simulink model "PART2"  (R2018b)
settings: Solver=ode2  StartTime=0.0  StopTime=500  FixedStep=0.1  RelTol=1e-3
settings Model: Creator=HP  LastModifiedBy=swastik

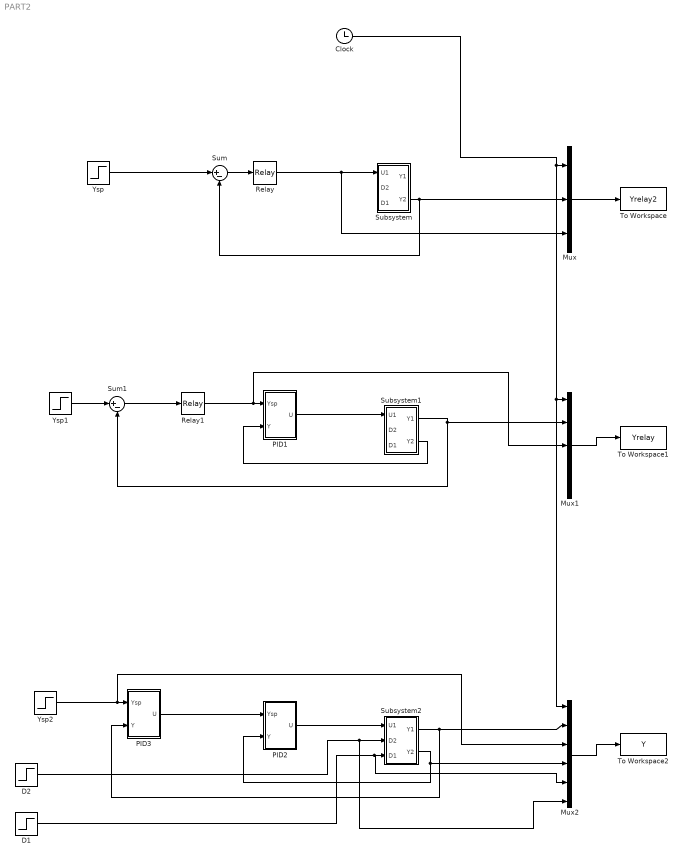
== system PART2 ==
  Clock : Clock
  D1 : Step  Time=0  After=0  SampleTime=0
  D2 : Step  Time=0  SampleTime=0
  Mux : Mux  Inputs=3
  Mux1 : Mux  Inputs=5
  Mux2 : Mux  Inputs=6
  PID1 : Subsystem  mask{Kc=1.6804/1.7, Ti=31.9/2, Td=31.9/8}
      mask prompts: Kc "Proportional Gain"; Ti "Integral time"; Td "Derivative time"
  PID2 : Subsystem  mask{Kc=1.6804/1.7, Ti=31.9/2, Td=31.9/8}
      mask prompts: Kc "Proportional Gain"; Ti "Integral time"; Td "Derivative time"
  PID3 : Subsystem  mask{Kc=2.0073/1.7, Ti=89.1/2, Td=89.1/8}
      mask prompts: Kc "Proportional Gain"; Ti "Integral time"; Td "Derivative time"
  Relay : Relay  OffOutputValue=-1
  Relay1 : Relay  OffOutputValue=-1
  Subsystem : Subsystem
  Subsystem1 : Subsystem
  Subsystem2 : Subsystem
  Sum : Sum  Inputs=|+-
  Sum1 : Sum  Inputs=|+-
  To Workspace : ToWorkspace  VariableName=Yrelay2  SampleTime=-1
  To Workspace1 : ToWorkspace  VariableName=Yrelay  SampleTime=-1
  To Workspace2 : ToWorkspace  VariableName=Y  SampleTime=-1
  Ysp : Step  Time=0  After=0  SampleTime=0
  Ysp1 : Step  Time=0  After=0  SampleTime=0
  Ysp2 : Step  Time=0  After=0  SampleTime=0
  wires:
  Ysp/1 -> Sum/1
  Sum/1 -> Relay/1
  Relay/1 -> Subsystem/1(U1), Mux/3
  Mux/1 -> To Workspace/1
  Clock/1 -> Mux2/1, Mux1/1, Mux/1
  Mux1/1 -> To Workspace1/1
  Subsystem/2(Y2) -> Mux/2, Sum/2
  PID1/1(U) -> Subsystem1/1(U1)
  Subsystem1/2(Y2) -> PID1/2(Y)
  Relay1/1 -> Mux1/3, PID1/1(Ysp)
  Sum1/1 -> Relay1/1
  Ysp1/1 -> Sum1/1
  Subsystem1/1(Y1) -> Mux1/2, Sum1/2
  Mux2/1 -> To Workspace2/1
  Subsystem2/2(Y2) -> Mux2/4, PID2/2(Y)
  PID2/1(U) -> Subsystem2/1(U1)
  Subsystem2/1(Y1) -> Mux2/2, PID3/2(Y)
  PID3/1(U) -> PID2/1(Ysp)
  Ysp2/1 -> Mux2/3, PID3/1(Ysp)
  D1/1 -> Mux2/5, Subsystem2/3(D1)
  D2/1 -> Mux2/6, Subsystem2/2(D2)

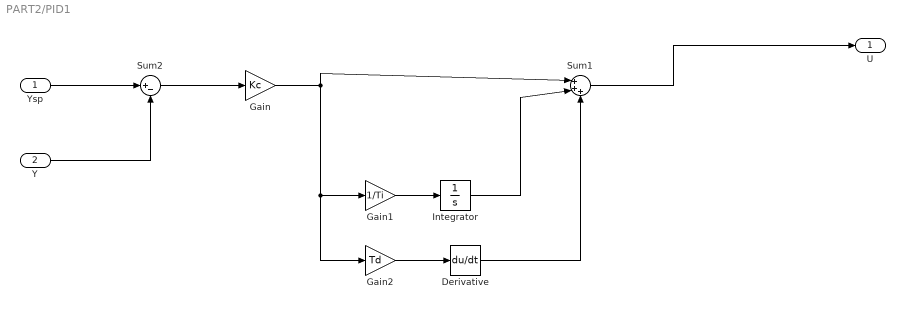
== system PART2/PID1 ==
  Ysp : Inport
  Y : Inport  Port=2
  Derivative : Derivative
  Gain : Gain  Gain=Kc
  Gain1 : Gain  Gain=1/Ti
  Gain2 : Gain  Gain=Td
  Integrator : Integrator
  Sum1 : Sum  Inputs=|+++
  Sum2 : Sum  Inputs=|+-
  U : Outport
  wires:
  Integrator/1 -> Sum1/2
  Gain/1 -> Sum1/1, Gain1/1, Gain2/1
  Sum2/1 -> Gain/1
  Y/1 -> Sum2/2
  Gain1/1 -> Integrator/1
  Gain2/1 -> Derivative/1
  Derivative/1 -> Sum1/3
  Ysp/1 -> Sum2/1
  Sum1/1 -> U/1

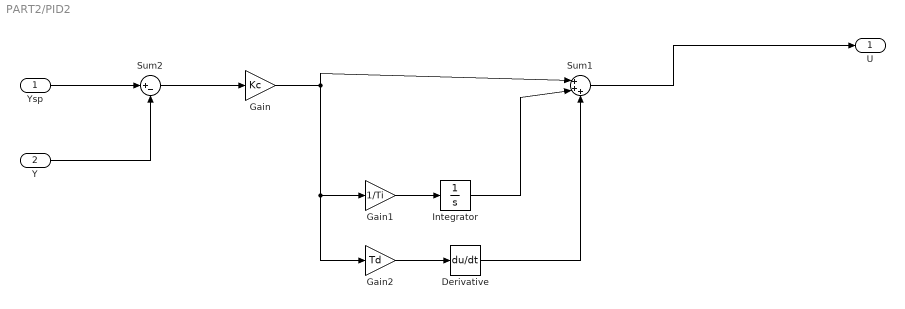
== system PART2/PID2 ==
  Ysp : Inport
  Y : Inport  Port=2
  Derivative : Derivative
  Gain : Gain  Gain=Kc
  Gain1 : Gain  Gain=1/Ti
  Gain2 : Gain  Gain=Td
  Integrator : Integrator
  Sum1 : Sum  Inputs=|+++
  Sum2 : Sum  Inputs=|+-
  U : Outport
  wires:
  Integrator/1 -> Sum1/2
  Gain/1 -> Sum1/1, Gain1/1, Gain2/1
  Sum2/1 -> Gain/1
  Y/1 -> Sum2/2
  Gain1/1 -> Integrator/1
  Gain2/1 -> Derivative/1
  Derivative/1 -> Sum1/3
  Ysp/1 -> Sum2/1
  Sum1/1 -> U/1

== system PART2/PID3 ==
  Ysp : Inport
  Y : Inport  Port=2
  Derivative : Derivative
  Gain : Gain  Gain=Kc
  Gain1 : Gain  Gain=1/Ti
  Gain2 : Gain  Gain=Td
  Integrator : Integrator
  Sum1 : Sum  Inputs=|+++
  Sum2 : Sum  Inputs=|+-
  U : Outport
  wires:
  Integrator/1 -> Sum1/2
  Gain/1 -> Sum1/1, Gain1/1, Gain2/1
  Sum2/1 -> Gain/1
  Y/1 -> Sum2/2
  Gain1/1 -> Integrator/1
  Gain2/1 -> Derivative/1
  Derivative/1 -> Sum1/3
  Ysp/1 -> Sum2/1
  Sum1/1 -> U/1

== system PART2/Subsystem ==
  U1 : Inport
  D2 : Inport  Port=2
  D1 : Inport  Port=3
  Process : Subsystem
  Y1 : Outport
  Y2 : Outport  Port=2
  wires:
  U1/1 -> Process/1(U)
  D2/1 -> Process/2(D2)
  D1/1 -> Process/3(D1)
  Process/1(Y1) -> Y1/1
  Process/2(Y2) -> Y2/1

== system PART2/Subsystem1 ==
  U1 : Inport
  D2 : Inport  Port=2
  D1 : Inport  Port=3
  Process : Subsystem
  Y1 : Outport
  Y2 : Outport  Port=2
  wires:
  U1/1 -> Process/1(U)
  D2/1 -> Process/2(D2)
  D1/1 -> Process/3(D1)
  Process/1(Y1) -> Y1/1
  Process/2(Y2) -> Y2/1

== system PART2/Subsystem2 ==
  U1 : Inport
  D2 : Inport  Port=2
  D1 : Inport  Port=3
  Process : Subsystem
  Y1 : Outport
  Y2 : Outport  Port=2
  wires:
  U1/1 -> Process/1(U)
  D2/1 -> Process/2(D2)
  D1/1 -> Process/3(D1)
  Process/1(Y1) -> Y1/1
  Process/2(Y2) -> Y2/1

== system PART2/Subsystem/Process ==
  U : Inport
  D2 : Inport  Port=2
  D1 : Inport  Port=3
  G1 : Subsystem  mask{K1=0.45, K2=0.45, T1=0.3, T2=0.3, K=1/17e-4}
      mask prompts: K1 "Forward Gain"; K2 "Rev Gain"; T1 "Forward Time Constt"; T2 "Rev Time Constt"; K "Scaling Gain"
  G2 : Subsystem  mask{K1=0.45, K2=0.45, T1=0.15, T2=0.15, K=2.01/17e-4}
      mask prompts: K1 "Forward Gain"; K2 "Rev Gain"; T1 "Forward Time Constt"; T2 "Rev Time Constt"; K "Scaling Gain"
  GD1 : Subsystem  mask{K1=0.45, K2=0.45, T1=0.1, T2=0.1, K=-1.005/17e-4}
      mask prompts: K1 "Forward Gain"; K2 "Rev Gain"; T1 "Forward Time Constt"; T2 "Rev Time Constt"; K "Scaling Gain"
  Sum : Sum  Inputs=|++
  Sum1 : Sum  Inputs=|++
  Y1 : Outport
  Y2 : Outport  Port=2
  wires:
  G1/1(Y) -> Sum1/1
  Sum/1 -> Y2/1, G1/1(U)
  G2/1(Y) -> Sum/1
  GD1/1(Y) -> Sum1/2
  U/1 -> G2/1(U)
  D1/1 -> GD1/1(U)
  D2/1 -> Sum/2
  Sum1/1 -> Y1/1

== system PART2/Subsystem1/Process ==
  U : Inport
  D2 : Inport  Port=2
  D1 : Inport  Port=3
  G1 : Subsystem  mask{K1=0.45, K2=0.45, T1=0.3, T2=0.3, K=1/17e-4}
      mask prompts: K1 "Forward Gain"; K2 "Rev Gain"; T1 "Forward Time Constt"; T2 "Rev Time Constt"; K "Scaling Gain"
  G2 : Subsystem  mask{K1=0.45, K2=0.45, T1=0.15, T2=0.15, K=2.01/17e-4}
      mask prompts: K1 "Forward Gain"; K2 "Rev Gain"; T1 "Forward Time Constt"; T2 "Rev Time Constt"; K "Scaling Gain"
  GD1 : Subsystem  mask{K1=0.45, K2=0.45, T1=0.1, T2=0.1, K=-1.005/17e-4}
      mask prompts: K1 "Forward Gain"; K2 "Rev Gain"; T1 "Forward Time Constt"; T2 "Rev Time Constt"; K "Scaling Gain"
  Sum : Sum  Inputs=|++
  Sum1 : Sum  Inputs=|++
  Y1 : Outport
  Y2 : Outport  Port=2
  wires:
  G1/1(Y) -> Sum1/1
  Sum/1 -> Y2/1, G1/1(U)
  G2/1(Y) -> Sum/1
  GD1/1(Y) -> Sum1/2
  U/1 -> G2/1(U)
  D1/1 -> GD1/1(U)
  D2/1 -> Sum/2
  Sum1/1 -> Y1/1

== system PART2/Subsystem2/Process ==
  U : Inport
  D2 : Inport  Port=2
  D1 : Inport  Port=3
  G1 : Subsystem  mask{K1=0.45, K2=0.45, T1=0.3, T2=0.3, K=1/17e-4}
      mask prompts: K1 "Forward Gain"; K2 "Rev Gain"; T1 "Forward Time Constt"; T2 "Rev Time Constt"; K "Scaling Gain"
  G2 : Subsystem  mask{K1=0.45, K2=0.45, T1=0.15, T2=0.15, K=2.01/17e-4}
      mask prompts: K1 "Forward Gain"; K2 "Rev Gain"; T1 "Forward Time Constt"; T2 "Rev Time Constt"; K "Scaling Gain"
  GD1 : Subsystem  mask{K1=0.45, K2=0.45, T1=0.1, T2=0.1, K=-1.005/17e-4}
      mask prompts: K1 "Forward Gain"; K2 "Rev Gain"; T1 "Forward Time Constt"; T2 "Rev Time Constt"; K "Scaling Gain"
  Sum : Sum  Inputs=|++
  Sum1 : Sum  Inputs=|++
  Y1 : Outport
  Y2 : Outport  Port=2
  wires:
  G1/1(Y) -> Sum1/1
  Sum/1 -> Y2/1, G1/1(U)
  G2/1(Y) -> Sum/1
  GD1/1(Y) -> Sum1/2
  U/1 -> G2/1(U)
  D1/1 -> GD1/1(U)
  D2/1 -> Sum/2
  Sum1/1 -> Y1/1

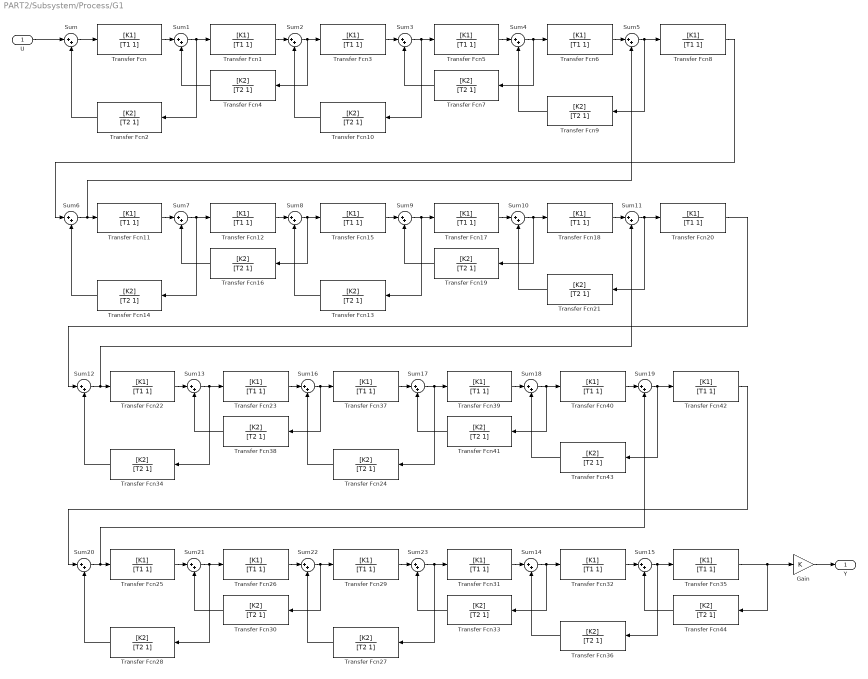
== system PART2/Subsystem/Process/G1 ==
  U : Inport
  Gain : Gain  Gain=K
  Sum{,1..23} (24 alike) : Sum  Inputs=|++
  Transfer Fcn{,1,3,5..6,8,11..12,15,17..18,20,22..23,25..26,29,31..32,35,37,39..40,42} (24 alike) : TransferFcn  Numerator=[K1]  Denominator=[T1 1]
  Transfer Fcn{2,4,7,9..10,13..14,16,19,21,24,27..28,30,33..34,36,38,41,43..44} (21 alike) : TransferFcn  Numerator=[K2]  Denominator=[T2 1]
  Y : Outport
  wires:
  Transfer Fcn14/1 -> Sum6/2
  Transfer Fcn13/1 -> Sum8/2
  Transfer Fcn18/1 -> Sum11/1
  Transfer Fcn1/1 -> Sum2/1
  Sum18/1 -> Transfer Fcn41/1, Transfer Fcn40/1
  Sum21/1 -> Transfer Fcn28/1, Transfer Fcn26/1
  Transfer Fcn26/1 -> Sum22/1
  Transfer Fcn15/1 -> Sum9/1
  Sum13/1 -> Transfer Fcn34/1, Transfer Fcn23/1
  Sum7/1 -> Transfer Fcn14/1, Transfer Fcn12/1
  Sum8/1 -> Transfer Fcn16/1, Transfer Fcn15/1
  Transfer Fcn20/1 -> Sum12/1
  Sum20/1 -> Sum19/2, Transfer Fcn25/1
  Transfer Fcn9/1 -> Sum4/2
  Transfer Fcn25/1 -> Sum21/1
  Sum12/1 -> Sum11/2, Transfer Fcn22/1
  Transfer Fcn12/1 -> Sum8/1
  Transfer Fcn16/1 -> Sum7/2
  Transfer Fcn44/1 -> Sum15/2
  Transfer Fcn39/1 -> Sum18/1
  Sum2/1 -> Transfer Fcn4/1, Transfer Fcn3/1
  Transfer Fcn38/1 -> Sum13/2
  Sum17/1 -> Transfer Fcn24/1, Transfer Fcn39/1
  Sum9/1 -> Transfer Fcn13/1, Transfer Fcn17/1
  Transfer Fcn35/1 -> Gain/1, Transfer Fcn44/1
  Sum11/1 -> Transfer Fcn21/1, Transfer Fcn20/1
  Transfer Fcn42/1 -> Sum20/1
  Sum1/1 -> Transfer Fcn2/1, Transfer Fcn1/1
  Sum15/1 -> Transfer Fcn36/1, Transfer Fcn35/1
  Transfer Fcn27/1 -> Sum22/2
  Transfer Fcn24/1 -> Sum16/2
  Transfer Fcn31/1 -> Sum14/1
  Transfer Fcn23/1 -> Sum16/1
  Sum14/1 -> Transfer Fcn33/1, Transfer Fcn32/1
  Sum23/1 -> Transfer Fcn27/1, Transfer Fcn31/1
  Transfer Fcn40/1 -> Sum19/1
  Sum16/1 -> Transfer Fcn38/1, Transfer Fcn37/1
  Transfer Fcn22/1 -> Sum13/1
  Transfer Fcn34/1 -> Sum12/2
  Transfer Fcn37/1 -> Sum17/1
  Transfer Fcn33/1 -> Sum23/2
  Transfer Fcn41/1 -> Sum17/2
  Sum4/1 -> Transfer Fcn7/1, Transfer Fcn6/1
  Transfer Fcn36/1 -> Sum14/2
  Sum10/1 -> Transfer Fcn19/1, Transfer Fcn18/1
  Sum22/1 -> Transfer Fcn30/1, Transfer Fcn29/1
  Transfer Fcn6/1 -> Sum5/1
  Transfer Fcn29/1 -> Sum23/1
  Transfer Fcn2/1 -> Sum/2
  Transfer Fcn28/1 -> Sum20/2
  Transfer Fcn17/1 -> Sum10/1
  Transfer Fcn30/1 -> Sum21/2
  Transfer Fcn43/1 -> Sum18/2
  Transfer Fcn5/1 -> Sum4/1
  Sum19/1 -> Transfer Fcn43/1, Transfer Fcn42/1
  Sum3/1 -> Transfer Fcn10/1, Transfer Fcn5/1
  Transfer Fcn32/1 -> Sum15/1
  Sum6/1 -> Sum5/2, Transfer Fcn11/1
  Transfer Fcn/1 -> Sum1/1
  Transfer Fcn21/1 -> Sum10/2
  Sum5/1 -> Transfer Fcn9/1, Transfer Fcn8/1
  Transfer Fcn7/1 -> Sum3/2
  Transfer Fcn4/1 -> Sum1/2
  Transfer Fcn11/1 -> Sum7/1
  Transfer Fcn10/1 -> Sum2/2
  Transfer Fcn3/1 -> Sum3/1
  Transfer Fcn8/1 -> Sum6/1
  Transfer Fcn19/1 -> Sum9/2
  Sum/1 -> Transfer Fcn/1
  Gain/1 -> Y/1
  U/1 -> Sum/1

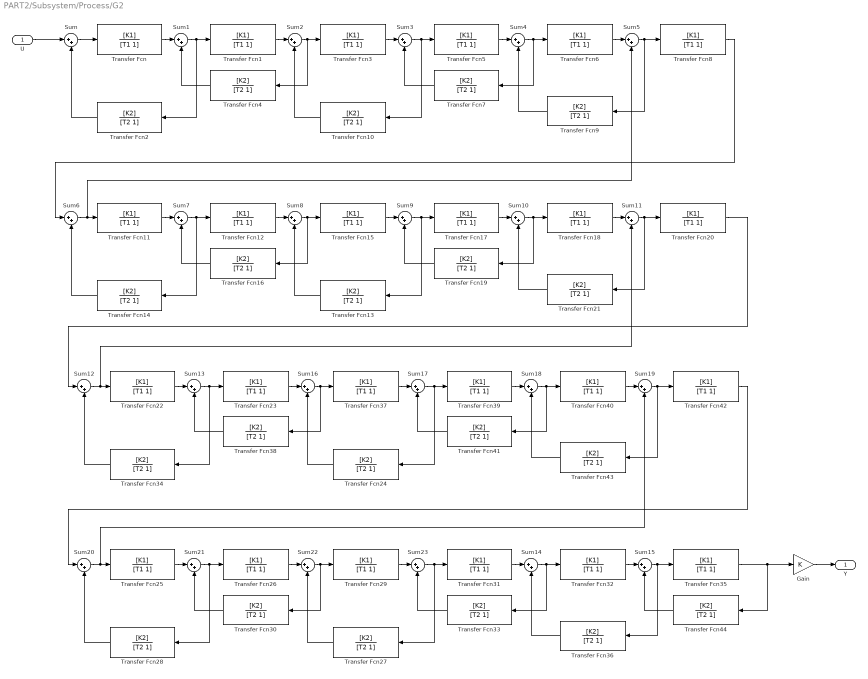
== system PART2/Subsystem/Process/G2 ==
  U : Inport
  Gain : Gain  Gain=K
  Sum{,1..23} (24 alike) : Sum  Inputs=|++
  Transfer Fcn{,1,3,5..6,8,11..12,15,17..18,20,22..23,25..26,29,31..32,35,37,39..40,42} (24 alike) : TransferFcn  Numerator=[K1]  Denominator=[T1 1]
  Transfer Fcn{2,4,7,9..10,13..14,16,19,21,24,27..28,30,33..34,36,38,41,43..44} (21 alike) : TransferFcn  Numerator=[K2]  Denominator=[T2 1]
  Y : Outport
  wires:
  Transfer Fcn14/1 -> Sum6/2
  Transfer Fcn13/1 -> Sum8/2
  Transfer Fcn18/1 -> Sum11/1
  Transfer Fcn1/1 -> Sum2/1
  Sum18/1 -> Transfer Fcn41/1, Transfer Fcn40/1
  Sum21/1 -> Transfer Fcn28/1, Transfer Fcn26/1
  Transfer Fcn26/1 -> Sum22/1
  Transfer Fcn15/1 -> Sum9/1
  Sum13/1 -> Transfer Fcn34/1, Transfer Fcn23/1
  Sum7/1 -> Transfer Fcn14/1, Transfer Fcn12/1
  Sum8/1 -> Transfer Fcn16/1, Transfer Fcn15/1
  Transfer Fcn20/1 -> Sum12/1
  Sum20/1 -> Sum19/2, Transfer Fcn25/1
  Transfer Fcn9/1 -> Sum4/2
  Transfer Fcn25/1 -> Sum21/1
  Sum12/1 -> Sum11/2, Transfer Fcn22/1
  Transfer Fcn12/1 -> Sum8/1
  Transfer Fcn16/1 -> Sum7/2
  Transfer Fcn44/1 -> Sum15/2
  Transfer Fcn39/1 -> Sum18/1
  Sum2/1 -> Transfer Fcn4/1, Transfer Fcn3/1
  Transfer Fcn38/1 -> Sum13/2
  Sum17/1 -> Transfer Fcn24/1, Transfer Fcn39/1
  Sum9/1 -> Transfer Fcn13/1, Transfer Fcn17/1
  Transfer Fcn35/1 -> Gain/1, Transfer Fcn44/1
  Sum11/1 -> Transfer Fcn21/1, Transfer Fcn20/1
  Transfer Fcn42/1 -> Sum20/1
  Sum1/1 -> Transfer Fcn2/1, Transfer Fcn1/1
  Sum15/1 -> Transfer Fcn36/1, Transfer Fcn35/1
  Transfer Fcn27/1 -> Sum22/2
  Transfer Fcn24/1 -> Sum16/2
  Transfer Fcn31/1 -> Sum14/1
  Transfer Fcn23/1 -> Sum16/1
  Sum14/1 -> Transfer Fcn33/1, Transfer Fcn32/1
  Sum23/1 -> Transfer Fcn27/1, Transfer Fcn31/1
  Transfer Fcn40/1 -> Sum19/1
  Sum16/1 -> Transfer Fcn38/1, Transfer Fcn37/1
  Transfer Fcn22/1 -> Sum13/1
  Transfer Fcn34/1 -> Sum12/2
  Transfer Fcn37/1 -> Sum17/1
  Transfer Fcn33/1 -> Sum23/2
  Transfer Fcn41/1 -> Sum17/2
  Sum4/1 -> Transfer Fcn7/1, Transfer Fcn6/1
  Transfer Fcn36/1 -> Sum14/2
  Sum10/1 -> Transfer Fcn19/1, Transfer Fcn18/1
  Sum22/1 -> Transfer Fcn30/1, Transfer Fcn29/1
  Transfer Fcn6/1 -> Sum5/1
  Transfer Fcn29/1 -> Sum23/1
  Transfer Fcn2/1 -> Sum/2
  Transfer Fcn28/1 -> Sum20/2
  Transfer Fcn17/1 -> Sum10/1
  Transfer Fcn30/1 -> Sum21/2
  Transfer Fcn43/1 -> Sum18/2
  Transfer Fcn5/1 -> Sum4/1
  Sum19/1 -> Transfer Fcn43/1, Transfer Fcn42/1
  Sum3/1 -> Transfer Fcn10/1, Transfer Fcn5/1
  Transfer Fcn32/1 -> Sum15/1
  Sum6/1 -> Sum5/2, Transfer Fcn11/1
  Transfer Fcn/1 -> Sum1/1
  Transfer Fcn21/1 -> Sum10/2
  Sum5/1 -> Transfer Fcn9/1, Transfer Fcn8/1
  Transfer Fcn7/1 -> Sum3/2
  Transfer Fcn4/1 -> Sum1/2
  Transfer Fcn11/1 -> Sum7/1
  Transfer Fcn10/1 -> Sum2/2
  Transfer Fcn3/1 -> Sum3/1
  Transfer Fcn8/1 -> Sum6/1
  Transfer Fcn19/1 -> Sum9/2
  Sum/1 -> Transfer Fcn/1
  Gain/1 -> Y/1
  U/1 -> Sum/1

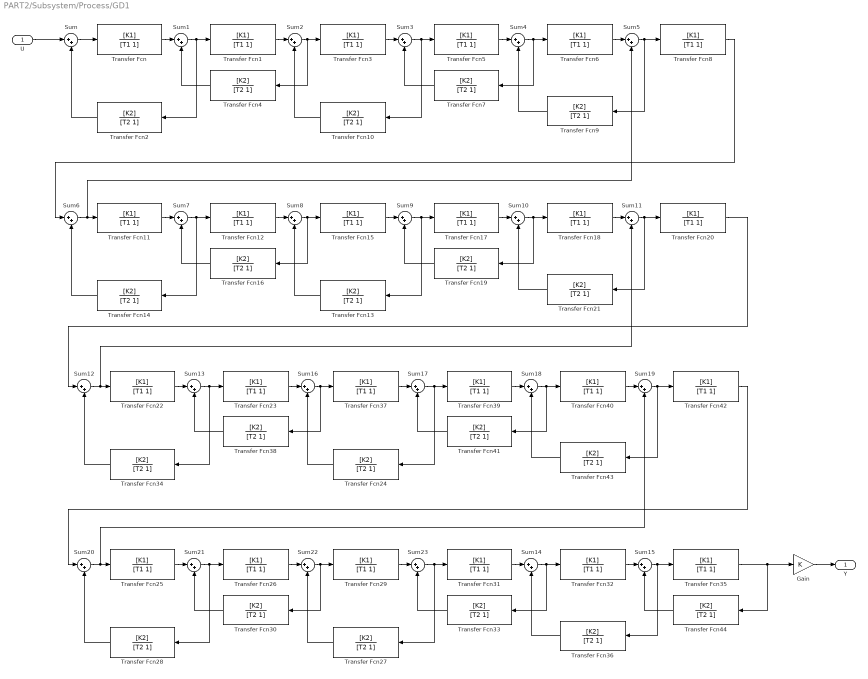
== system PART2/Subsystem/Process/GD1 ==
  U : Inport
  Gain : Gain  Gain=K
  Sum{,1..23} (24 alike) : Sum  Inputs=|++
  Transfer Fcn{,1,3,5..6,8,11..12,15,17..18,20,22..23,25..26,29,31..32,35,37,39..40,42} (24 alike) : TransferFcn  Numerator=[K1]  Denominator=[T1 1]
  Transfer Fcn{2,4,7,9..10,13..14,16,19,21,24,27..28,30,33..34,36,38,41,43..44} (21 alike) : TransferFcn  Numerator=[K2]  Denominator=[T2 1]
  Y : Outport
  wires:
  Transfer Fcn14/1 -> Sum6/2
  Transfer Fcn13/1 -> Sum8/2
  Transfer Fcn18/1 -> Sum11/1
  Transfer Fcn1/1 -> Sum2/1
  Sum18/1 -> Transfer Fcn41/1, Transfer Fcn40/1
  Sum21/1 -> Transfer Fcn28/1, Transfer Fcn26/1
  Transfer Fcn26/1 -> Sum22/1
  Transfer Fcn15/1 -> Sum9/1
  Sum13/1 -> Transfer Fcn34/1, Transfer Fcn23/1
  Sum7/1 -> Transfer Fcn14/1, Transfer Fcn12/1
  Sum8/1 -> Transfer Fcn16/1, Transfer Fcn15/1
  Transfer Fcn20/1 -> Sum12/1
  Sum20/1 -> Sum19/2, Transfer Fcn25/1
  Transfer Fcn9/1 -> Sum4/2
  Transfer Fcn25/1 -> Sum21/1
  Sum12/1 -> Sum11/2, Transfer Fcn22/1
  Transfer Fcn12/1 -> Sum8/1
  Transfer Fcn16/1 -> Sum7/2
  Transfer Fcn44/1 -> Sum15/2
  Transfer Fcn39/1 -> Sum18/1
  Sum2/1 -> Transfer Fcn4/1, Transfer Fcn3/1
  Transfer Fcn38/1 -> Sum13/2
  Sum17/1 -> Transfer Fcn24/1, Transfer Fcn39/1
  Sum9/1 -> Transfer Fcn13/1, Transfer Fcn17/1
  Transfer Fcn35/1 -> Gain/1, Transfer Fcn44/1
  Sum11/1 -> Transfer Fcn21/1, Transfer Fcn20/1
  Transfer Fcn42/1 -> Sum20/1
  Sum1/1 -> Transfer Fcn2/1, Transfer Fcn1/1
  Sum15/1 -> Transfer Fcn36/1, Transfer Fcn35/1
  Transfer Fcn27/1 -> Sum22/2
  Transfer Fcn24/1 -> Sum16/2
  Transfer Fcn31/1 -> Sum14/1
  Transfer Fcn23/1 -> Sum16/1
  Sum14/1 -> Transfer Fcn33/1, Transfer Fcn32/1
  Sum23/1 -> Transfer Fcn27/1, Transfer Fcn31/1
  Transfer Fcn40/1 -> Sum19/1
  Sum16/1 -> Transfer Fcn38/1, Transfer Fcn37/1
  Transfer Fcn22/1 -> Sum13/1
  Transfer Fcn34/1 -> Sum12/2
  Transfer Fcn37/1 -> Sum17/1
  Transfer Fcn33/1 -> Sum23/2
  Transfer Fcn41/1 -> Sum17/2
  Sum4/1 -> Transfer Fcn7/1, Transfer Fcn6/1
  Transfer Fcn36/1 -> Sum14/2
  Sum10/1 -> Transfer Fcn19/1, Transfer Fcn18/1
  Sum22/1 -> Transfer Fcn30/1, Transfer Fcn29/1
  Transfer Fcn6/1 -> Sum5/1
  Transfer Fcn29/1 -> Sum23/1
  Transfer Fcn2/1 -> Sum/2
  Transfer Fcn28/1 -> Sum20/2
  Transfer Fcn17/1 -> Sum10/1
  Transfer Fcn30/1 -> Sum21/2
  Transfer Fcn43/1 -> Sum18/2
  Transfer Fcn5/1 -> Sum4/1
  Sum19/1 -> Transfer Fcn43/1, Transfer Fcn42/1
  Sum3/1 -> Transfer Fcn10/1, Transfer Fcn5/1
  Transfer Fcn32/1 -> Sum15/1
  Sum6/1 -> Sum5/2, Transfer Fcn11/1
  Transfer Fcn/1 -> Sum1/1
  Transfer Fcn21/1 -> Sum10/2
  Sum5/1 -> Transfer Fcn9/1, Transfer Fcn8/1
  Transfer Fcn7/1 -> Sum3/2
  Transfer Fcn4/1 -> Sum1/2
  Transfer Fcn11/1 -> Sum7/1
  Transfer Fcn10/1 -> Sum2/2
  Transfer Fcn3/1 -> Sum3/1
  Transfer Fcn8/1 -> Sum6/1
  Transfer Fcn19/1 -> Sum9/2
  Sum/1 -> Transfer Fcn/1
  Gain/1 -> Y/1
  U/1 -> Sum/1

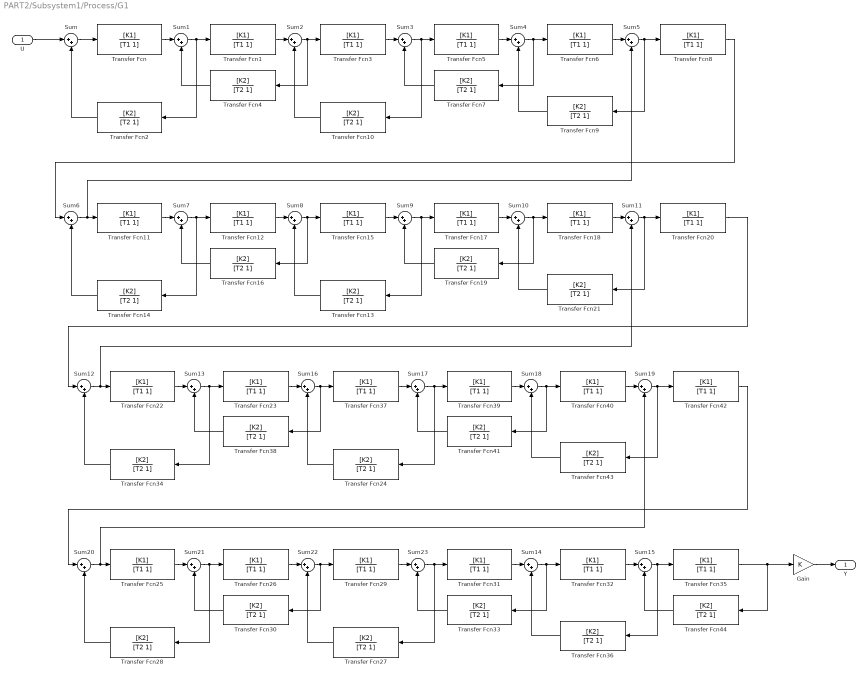
== system PART2/Subsystem1/Process/G1 ==
  U : Inport
  Gain : Gain  Gain=K
  Sum{,1..23} (24 alike) : Sum  Inputs=|++
  Transfer Fcn{,1,3,5..6,8,11..12,15,17..18,20,22..23,25..26,29,31..32,35,37,39..40,42} (24 alike) : TransferFcn  Numerator=[K1]  Denominator=[T1 1]
  Transfer Fcn{2,4,7,9..10,13..14,16,19,21,24,27..28,30,33..34,36,38,41,43..44} (21 alike) : TransferFcn  Numerator=[K2]  Denominator=[T2 1]
  Y : Outport
  wires:
  Transfer Fcn14/1 -> Sum6/2
  Transfer Fcn13/1 -> Sum8/2
  Transfer Fcn18/1 -> Sum11/1
  Transfer Fcn1/1 -> Sum2/1
  Sum18/1 -> Transfer Fcn41/1, Transfer Fcn40/1
  Sum21/1 -> Transfer Fcn28/1, Transfer Fcn26/1
  Transfer Fcn26/1 -> Sum22/1
  Transfer Fcn15/1 -> Sum9/1
  Sum13/1 -> Transfer Fcn34/1, Transfer Fcn23/1
  Sum7/1 -> Transfer Fcn14/1, Transfer Fcn12/1
  Sum8/1 -> Transfer Fcn16/1, Transfer Fcn15/1
  Transfer Fcn20/1 -> Sum12/1
  Sum20/1 -> Sum19/2, Transfer Fcn25/1
  Transfer Fcn9/1 -> Sum4/2
  Transfer Fcn25/1 -> Sum21/1
  Sum12/1 -> Sum11/2, Transfer Fcn22/1
  Transfer Fcn12/1 -> Sum8/1
  Transfer Fcn16/1 -> Sum7/2
  Transfer Fcn44/1 -> Sum15/2
  Transfer Fcn39/1 -> Sum18/1
  Sum2/1 -> Transfer Fcn4/1, Transfer Fcn3/1
  Transfer Fcn38/1 -> Sum13/2
  Sum17/1 -> Transfer Fcn24/1, Transfer Fcn39/1
  Sum9/1 -> Transfer Fcn13/1, Transfer Fcn17/1
  Transfer Fcn35/1 -> Gain/1, Transfer Fcn44/1
  Sum11/1 -> Transfer Fcn21/1, Transfer Fcn20/1
  Transfer Fcn42/1 -> Sum20/1
  Sum1/1 -> Transfer Fcn2/1, Transfer Fcn1/1
  Sum15/1 -> Transfer Fcn36/1, Transfer Fcn35/1
  Transfer Fcn27/1 -> Sum22/2
  Transfer Fcn24/1 -> Sum16/2
  Transfer Fcn31/1 -> Sum14/1
  Transfer Fcn23/1 -> Sum16/1
  Sum14/1 -> Transfer Fcn33/1, Transfer Fcn32/1
  Sum23/1 -> Transfer Fcn27/1, Transfer Fcn31/1
  Transfer Fcn40/1 -> Sum19/1
  Sum16/1 -> Transfer Fcn38/1, Transfer Fcn37/1
  Transfer Fcn22/1 -> Sum13/1
  Transfer Fcn34/1 -> Sum12/2
  Transfer Fcn37/1 -> Sum17/1
  Transfer Fcn33/1 -> Sum23/2
  Transfer Fcn41/1 -> Sum17/2
  Sum4/1 -> Transfer Fcn7/1, Transfer Fcn6/1
  Transfer Fcn36/1 -> Sum14/2
  Sum10/1 -> Transfer Fcn19/1, Transfer Fcn18/1
  Sum22/1 -> Transfer Fcn30/1, Transfer Fcn29/1
  Transfer Fcn6/1 -> Sum5/1
  Transfer Fcn29/1 -> Sum23/1
  Transfer Fcn2/1 -> Sum/2
  Transfer Fcn28/1 -> Sum20/2
  Transfer Fcn17/1 -> Sum10/1
  Transfer Fcn30/1 -> Sum21/2
  Transfer Fcn43/1 -> Sum18/2
  Transfer Fcn5/1 -> Sum4/1
  Sum19/1 -> Transfer Fcn43/1, Transfer Fcn42/1
  Sum3/1 -> Transfer Fcn10/1, Transfer Fcn5/1
  Transfer Fcn32/1 -> Sum15/1
  Sum6/1 -> Sum5/2, Transfer Fcn11/1
  Transfer Fcn/1 -> Sum1/1
  Transfer Fcn21/1 -> Sum10/2
  Sum5/1 -> Transfer Fcn9/1, Transfer Fcn8/1
  Transfer Fcn7/1 -> Sum3/2
  Transfer Fcn4/1 -> Sum1/2
  Transfer Fcn11/1 -> Sum7/1
  Transfer Fcn10/1 -> Sum2/2
  Transfer Fcn3/1 -> Sum3/1
  Transfer Fcn8/1 -> Sum6/1
  Transfer Fcn19/1 -> Sum9/2
  Sum/1 -> Transfer Fcn/1
  Gain/1 -> Y/1
  U/1 -> Sum/1

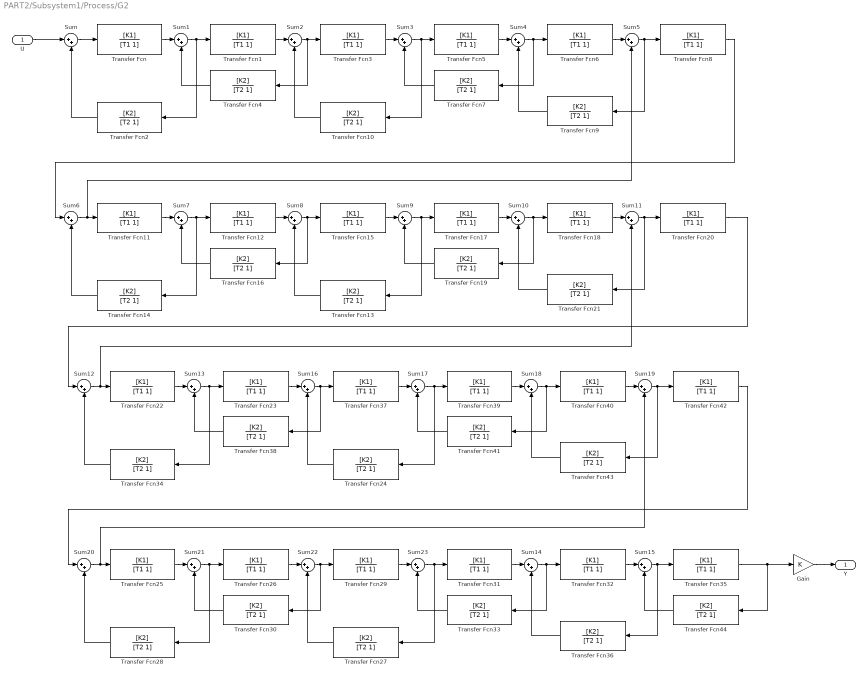
== system PART2/Subsystem1/Process/G2 ==
  U : Inport
  Gain : Gain  Gain=K
  Sum{,1..23} (24 alike) : Sum  Inputs=|++
  Transfer Fcn{,1,3,5..6,8,11..12,15,17..18,20,22..23,25..26,29,31..32,35,37,39..40,42} (24 alike) : TransferFcn  Numerator=[K1]  Denominator=[T1 1]
  Transfer Fcn{2,4,7,9..10,13..14,16,19,21,24,27..28,30,33..34,36,38,41,43..44} (21 alike) : TransferFcn  Numerator=[K2]  Denominator=[T2 1]
  Y : Outport
  wires:
  Transfer Fcn14/1 -> Sum6/2
  Transfer Fcn13/1 -> Sum8/2
  Transfer Fcn18/1 -> Sum11/1
  Transfer Fcn1/1 -> Sum2/1
  Sum18/1 -> Transfer Fcn41/1, Transfer Fcn40/1
  Sum21/1 -> Transfer Fcn28/1, Transfer Fcn26/1
  Transfer Fcn26/1 -> Sum22/1
  Transfer Fcn15/1 -> Sum9/1
  Sum13/1 -> Transfer Fcn34/1, Transfer Fcn23/1
  Sum7/1 -> Transfer Fcn14/1, Transfer Fcn12/1
  Sum8/1 -> Transfer Fcn16/1, Transfer Fcn15/1
  Transfer Fcn20/1 -> Sum12/1
  Sum20/1 -> Sum19/2, Transfer Fcn25/1
  Transfer Fcn9/1 -> Sum4/2
  Transfer Fcn25/1 -> Sum21/1
  Sum12/1 -> Sum11/2, Transfer Fcn22/1
  Transfer Fcn12/1 -> Sum8/1
  Transfer Fcn16/1 -> Sum7/2
  Transfer Fcn44/1 -> Sum15/2
  Transfer Fcn39/1 -> Sum18/1
  Sum2/1 -> Transfer Fcn4/1, Transfer Fcn3/1
  Transfer Fcn38/1 -> Sum13/2
  Sum17/1 -> Transfer Fcn24/1, Transfer Fcn39/1
  Sum9/1 -> Transfer Fcn13/1, Transfer Fcn17/1
  Transfer Fcn35/1 -> Gain/1, Transfer Fcn44/1
  Sum11/1 -> Transfer Fcn21/1, Transfer Fcn20/1
  Transfer Fcn42/1 -> Sum20/1
  Sum1/1 -> Transfer Fcn2/1, Transfer Fcn1/1
  Sum15/1 -> Transfer Fcn36/1, Transfer Fcn35/1
  Transfer Fcn27/1 -> Sum22/2
  Transfer Fcn24/1 -> Sum16/2
  Transfer Fcn31/1 -> Sum14/1
  Transfer Fcn23/1 -> Sum16/1
  Sum14/1 -> Transfer Fcn33/1, Transfer Fcn32/1
  Sum23/1 -> Transfer Fcn27/1, Transfer Fcn31/1
  Transfer Fcn40/1 -> Sum19/1
  Sum16/1 -> Transfer Fcn38/1, Transfer Fcn37/1
  Transfer Fcn22/1 -> Sum13/1
  Transfer Fcn34/1 -> Sum12/2
  Transfer Fcn37/1 -> Sum17/1
  Transfer Fcn33/1 -> Sum23/2
  Transfer Fcn41/1 -> Sum17/2
  Sum4/1 -> Transfer Fcn7/1, Transfer Fcn6/1
  Transfer Fcn36/1 -> Sum14/2
  Sum10/1 -> Transfer Fcn19/1, Transfer Fcn18/1
  Sum22/1 -> Transfer Fcn30/1, Transfer Fcn29/1
  Transfer Fcn6/1 -> Sum5/1
  Transfer Fcn29/1 -> Sum23/1
  Transfer Fcn2/1 -> Sum/2
  Transfer Fcn28/1 -> Sum20/2
  Transfer Fcn17/1 -> Sum10/1
  Transfer Fcn30/1 -> Sum21/2
  Transfer Fcn43/1 -> Sum18/2
  Transfer Fcn5/1 -> Sum4/1
  Sum19/1 -> Transfer Fcn43/1, Transfer Fcn42/1
  Sum3/1 -> Transfer Fcn10/1, Transfer Fcn5/1
  Transfer Fcn32/1 -> Sum15/1
  Sum6/1 -> Sum5/2, Transfer Fcn11/1
  Transfer Fcn/1 -> Sum1/1
  Transfer Fcn21/1 -> Sum10/2
  Sum5/1 -> Transfer Fcn9/1, Transfer Fcn8/1
  Transfer Fcn7/1 -> Sum3/2
  Transfer Fcn4/1 -> Sum1/2
  Transfer Fcn11/1 -> Sum7/1
  Transfer Fcn10/1 -> Sum2/2
  Transfer Fcn3/1 -> Sum3/1
  Transfer Fcn8/1 -> Sum6/1
  Transfer Fcn19/1 -> Sum9/2
  Sum/1 -> Transfer Fcn/1
  Gain/1 -> Y/1
  U/1 -> Sum/1

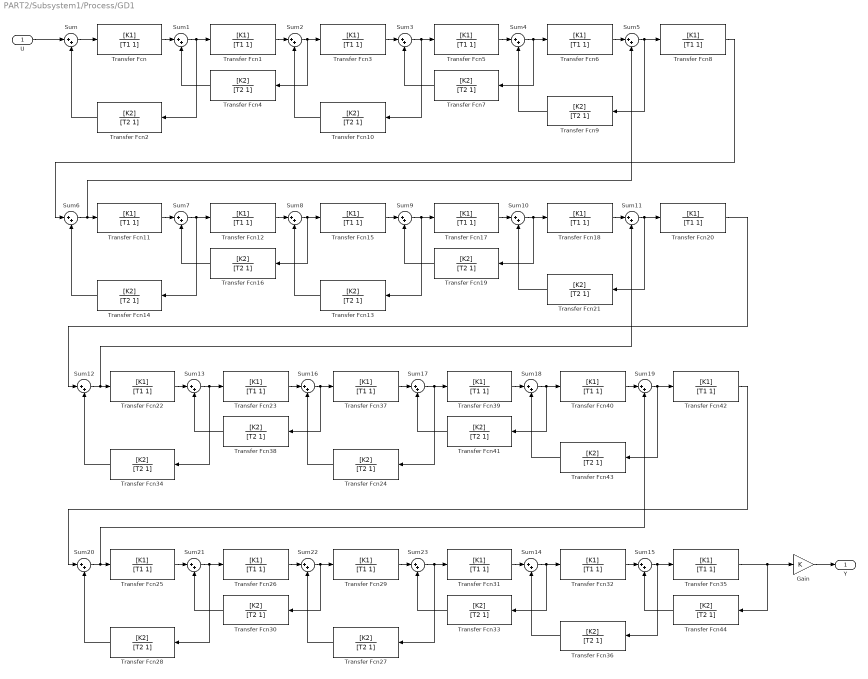
== system PART2/Subsystem1/Process/GD1 ==
  U : Inport
  Gain : Gain  Gain=K
  Sum{,1..23} (24 alike) : Sum  Inputs=|++
  Transfer Fcn{,1,3,5..6,8,11..12,15,17..18,20,22..23,25..26,29,31..32,35,37,39..40,42} (24 alike) : TransferFcn  Numerator=[K1]  Denominator=[T1 1]
  Transfer Fcn{2,4,7,9..10,13..14,16,19,21,24,27..28,30,33..34,36,38,41,43..44} (21 alike) : TransferFcn  Numerator=[K2]  Denominator=[T2 1]
  Y : Outport
  wires:
  Transfer Fcn14/1 -> Sum6/2
  Transfer Fcn13/1 -> Sum8/2
  Transfer Fcn18/1 -> Sum11/1
  Transfer Fcn1/1 -> Sum2/1
  Sum18/1 -> Transfer Fcn41/1, Transfer Fcn40/1
  Sum21/1 -> Transfer Fcn28/1, Transfer Fcn26/1
  Transfer Fcn26/1 -> Sum22/1
  Transfer Fcn15/1 -> Sum9/1
  Sum13/1 -> Transfer Fcn34/1, Transfer Fcn23/1
  Sum7/1 -> Transfer Fcn14/1, Transfer Fcn12/1
  Sum8/1 -> Transfer Fcn16/1, Transfer Fcn15/1
  Transfer Fcn20/1 -> Sum12/1
  Sum20/1 -> Sum19/2, Transfer Fcn25/1
  Transfer Fcn9/1 -> Sum4/2
  Transfer Fcn25/1 -> Sum21/1
  Sum12/1 -> Sum11/2, Transfer Fcn22/1
  Transfer Fcn12/1 -> Sum8/1
  Transfer Fcn16/1 -> Sum7/2
  Transfer Fcn44/1 -> Sum15/2
  Transfer Fcn39/1 -> Sum18/1
  Sum2/1 -> Transfer Fcn4/1, Transfer Fcn3/1
  Transfer Fcn38/1 -> Sum13/2
  Sum17/1 -> Transfer Fcn24/1, Transfer Fcn39/1
  Sum9/1 -> Transfer Fcn13/1, Transfer Fcn17/1
  Transfer Fcn35/1 -> Gain/1, Transfer Fcn44/1
  Sum11/1 -> Transfer Fcn21/1, Transfer Fcn20/1
  Transfer Fcn42/1 -> Sum20/1
  Sum1/1 -> Transfer Fcn2/1, Transfer Fcn1/1
  Sum15/1 -> Transfer Fcn36/1, Transfer Fcn35/1
  Transfer Fcn27/1 -> Sum22/2
  Transfer Fcn24/1 -> Sum16/2
  Transfer Fcn31/1 -> Sum14/1
  Transfer Fcn23/1 -> Sum16/1
  Sum14/1 -> Transfer Fcn33/1, Transfer Fcn32/1
  Sum23/1 -> Transfer Fcn27/1, Transfer Fcn31/1
  Transfer Fcn40/1 -> Sum19/1
  Sum16/1 -> Transfer Fcn38/1, Transfer Fcn37/1
  Transfer Fcn22/1 -> Sum13/1
  Transfer Fcn34/1 -> Sum12/2
  Transfer Fcn37/1 -> Sum17/1
  Transfer Fcn33/1 -> Sum23/2
  Transfer Fcn41/1 -> Sum17/2
  Sum4/1 -> Transfer Fcn7/1, Transfer Fcn6/1
  Transfer Fcn36/1 -> Sum14/2
  Sum10/1 -> Transfer Fcn19/1, Transfer Fcn18/1
  Sum22/1 -> Transfer Fcn30/1, Transfer Fcn29/1
  Transfer Fcn6/1 -> Sum5/1
  Transfer Fcn29/1 -> Sum23/1
  Transfer Fcn2/1 -> Sum/2
  Transfer Fcn28/1 -> Sum20/2
  Transfer Fcn17/1 -> Sum10/1
  Transfer Fcn30/1 -> Sum21/2
  Transfer Fcn43/1 -> Sum18/2
  Transfer Fcn5/1 -> Sum4/1
  Sum19/1 -> Transfer Fcn43/1, Transfer Fcn42/1
  Sum3/1 -> Transfer Fcn10/1, Transfer Fcn5/1
  Transfer Fcn32/1 -> Sum15/1
  Sum6/1 -> Sum5/2, Transfer Fcn11/1
  Transfer Fcn/1 -> Sum1/1
  Transfer Fcn21/1 -> Sum10/2
  Sum5/1 -> Transfer Fcn9/1, Transfer Fcn8/1
  Transfer Fcn7/1 -> Sum3/2
  Transfer Fcn4/1 -> Sum1/2
  Transfer Fcn11/1 -> Sum7/1
  Transfer Fcn10/1 -> Sum2/2
  Transfer Fcn3/1 -> Sum3/1
  Transfer Fcn8/1 -> Sum6/1
  Transfer Fcn19/1 -> Sum9/2
  Sum/1 -> Transfer Fcn/1
  Gain/1 -> Y/1
  U/1 -> Sum/1

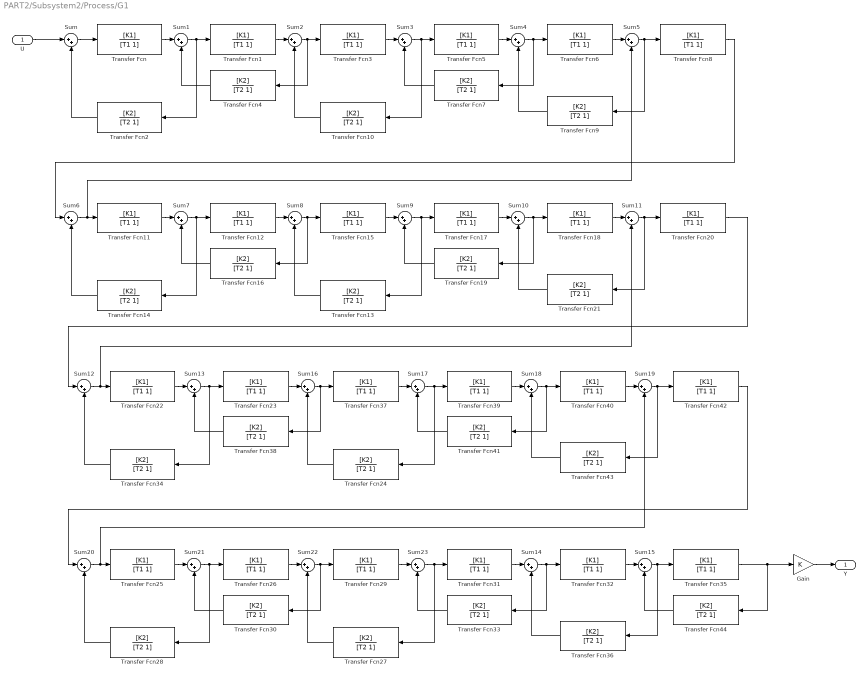
== system PART2/Subsystem2/Process/G1 ==
  U : Inport
  Gain : Gain  Gain=K
  Sum{,1..23} (24 alike) : Sum  Inputs=|++
  Transfer Fcn{,1,3,5..6,8,11..12,15,17..18,20,22..23,25..26,29,31..32,35,37,39..40,42} (24 alike) : TransferFcn  Numerator=[K1]  Denominator=[T1 1]
  Transfer Fcn{2,4,7,9..10,13..14,16,19,21,24,27..28,30,33..34,36,38,41,43..44} (21 alike) : TransferFcn  Numerator=[K2]  Denominator=[T2 1]
  Y : Outport
  wires:
  Transfer Fcn14/1 -> Sum6/2
  Transfer Fcn13/1 -> Sum8/2
  Transfer Fcn18/1 -> Sum11/1
  Transfer Fcn1/1 -> Sum2/1
  Sum18/1 -> Transfer Fcn41/1, Transfer Fcn40/1
  Sum21/1 -> Transfer Fcn28/1, Transfer Fcn26/1
  Transfer Fcn26/1 -> Sum22/1
  Transfer Fcn15/1 -> Sum9/1
  Sum13/1 -> Transfer Fcn34/1, Transfer Fcn23/1
  Sum7/1 -> Transfer Fcn14/1, Transfer Fcn12/1
  Sum8/1 -> Transfer Fcn16/1, Transfer Fcn15/1
  Transfer Fcn20/1 -> Sum12/1
  Sum20/1 -> Sum19/2, Transfer Fcn25/1
  Transfer Fcn9/1 -> Sum4/2
  Transfer Fcn25/1 -> Sum21/1
  Sum12/1 -> Sum11/2, Transfer Fcn22/1
  Transfer Fcn12/1 -> Sum8/1
  Transfer Fcn16/1 -> Sum7/2
  Transfer Fcn44/1 -> Sum15/2
  Transfer Fcn39/1 -> Sum18/1
  Sum2/1 -> Transfer Fcn4/1, Transfer Fcn3/1
  Transfer Fcn38/1 -> Sum13/2
  Sum17/1 -> Transfer Fcn24/1, Transfer Fcn39/1
  Sum9/1 -> Transfer Fcn13/1, Transfer Fcn17/1
  Transfer Fcn35/1 -> Gain/1, Transfer Fcn44/1
  Sum11/1 -> Transfer Fcn21/1, Transfer Fcn20/1
  Transfer Fcn42/1 -> Sum20/1
  Sum1/1 -> Transfer Fcn2/1, Transfer Fcn1/1
  Sum15/1 -> Transfer Fcn36/1, Transfer Fcn35/1
  Transfer Fcn27/1 -> Sum22/2
  Transfer Fcn24/1 -> Sum16/2
  Transfer Fcn31/1 -> Sum14/1
  Transfer Fcn23/1 -> Sum16/1
  Sum14/1 -> Transfer Fcn33/1, Transfer Fcn32/1
  Sum23/1 -> Transfer Fcn27/1, Transfer Fcn31/1
  Transfer Fcn40/1 -> Sum19/1
  Sum16/1 -> Transfer Fcn38/1, Transfer Fcn37/1
  Transfer Fcn22/1 -> Sum13/1
  Transfer Fcn34/1 -> Sum12/2
  Transfer Fcn37/1 -> Sum17/1
  Transfer Fcn33/1 -> Sum23/2
  Transfer Fcn41/1 -> Sum17/2
  Sum4/1 -> Transfer Fcn7/1, Transfer Fcn6/1
  Transfer Fcn36/1 -> Sum14/2
  Sum10/1 -> Transfer Fcn19/1, Transfer Fcn18/1
  Sum22/1 -> Transfer Fcn30/1, Transfer Fcn29/1
  Transfer Fcn6/1 -> Sum5/1
  Transfer Fcn29/1 -> Sum23/1
  Transfer Fcn2/1 -> Sum/2
  Transfer Fcn28/1 -> Sum20/2
  Transfer Fcn17/1 -> Sum10/1
  Transfer Fcn30/1 -> Sum21/2
  Transfer Fcn43/1 -> Sum18/2
  Transfer Fcn5/1 -> Sum4/1
  Sum19/1 -> Transfer Fcn43/1, Transfer Fcn42/1
  Sum3/1 -> Transfer Fcn10/1, Transfer Fcn5/1
  Transfer Fcn32/1 -> Sum15/1
  Sum6/1 -> Sum5/2, Transfer Fcn11/1
  Transfer Fcn/1 -> Sum1/1
  Transfer Fcn21/1 -> Sum10/2
  Sum5/1 -> Transfer Fcn9/1, Transfer Fcn8/1
  Transfer Fcn7/1 -> Sum3/2
  Transfer Fcn4/1 -> Sum1/2
  Transfer Fcn11/1 -> Sum7/1
  Transfer Fcn10/1 -> Sum2/2
  Transfer Fcn3/1 -> Sum3/1
  Transfer Fcn8/1 -> Sum6/1
  Transfer Fcn19/1 -> Sum9/2
  Sum/1 -> Transfer Fcn/1
  Gain/1 -> Y/1
  U/1 -> Sum/1

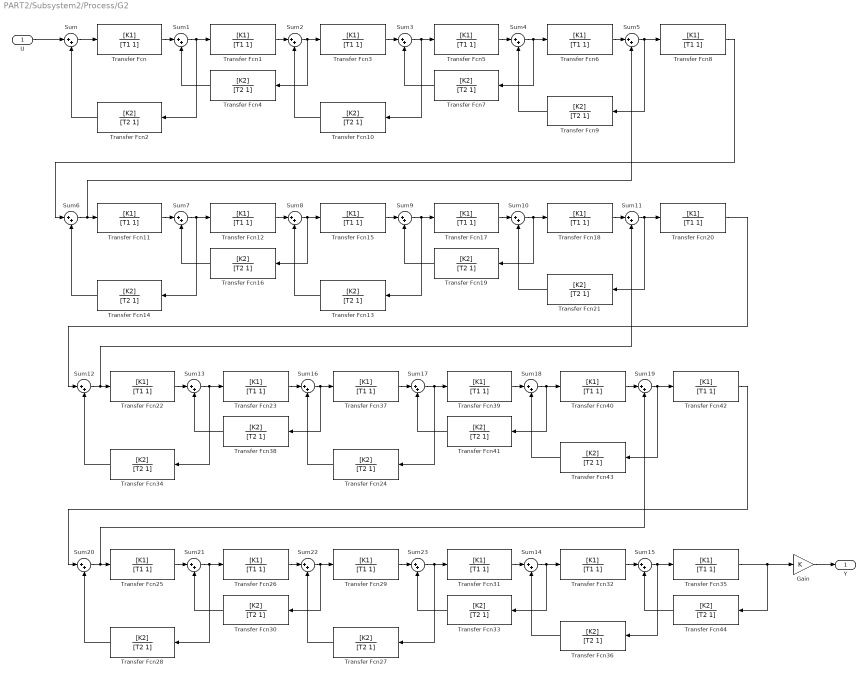
== system PART2/Subsystem2/Process/G2 ==
  U : Inport
  Gain : Gain  Gain=K
  Sum{,1..23} (24 alike) : Sum  Inputs=|++
  Transfer Fcn{,1,3,5..6,8,11..12,15,17..18,20,22..23,25..26,29,31..32,35,37,39..40,42} (24 alike) : TransferFcn  Numerator=[K1]  Denominator=[T1 1]
  Transfer Fcn{2,4,7,9..10,13..14,16,19,21,24,27..28,30,33..34,36,38,41,43..44} (21 alike) : TransferFcn  Numerator=[K2]  Denominator=[T2 1]
  Y : Outport
  wires:
  Transfer Fcn14/1 -> Sum6/2
  Transfer Fcn13/1 -> Sum8/2
  Transfer Fcn18/1 -> Sum11/1
  Transfer Fcn1/1 -> Sum2/1
  Sum18/1 -> Transfer Fcn41/1, Transfer Fcn40/1
  Sum21/1 -> Transfer Fcn28/1, Transfer Fcn26/1
  Transfer Fcn26/1 -> Sum22/1
  Transfer Fcn15/1 -> Sum9/1
  Sum13/1 -> Transfer Fcn34/1, Transfer Fcn23/1
  Sum7/1 -> Transfer Fcn14/1, Transfer Fcn12/1
  Sum8/1 -> Transfer Fcn16/1, Transfer Fcn15/1
  Transfer Fcn20/1 -> Sum12/1
  Sum20/1 -> Sum19/2, Transfer Fcn25/1
  Transfer Fcn9/1 -> Sum4/2
  Transfer Fcn25/1 -> Sum21/1
  Sum12/1 -> Sum11/2, Transfer Fcn22/1
  Transfer Fcn12/1 -> Sum8/1
  Transfer Fcn16/1 -> Sum7/2
  Transfer Fcn44/1 -> Sum15/2
  Transfer Fcn39/1 -> Sum18/1
  Sum2/1 -> Transfer Fcn4/1, Transfer Fcn3/1
  Transfer Fcn38/1 -> Sum13/2
  Sum17/1 -> Transfer Fcn24/1, Transfer Fcn39/1
  Sum9/1 -> Transfer Fcn13/1, Transfer Fcn17/1
  Transfer Fcn35/1 -> Gain/1, Transfer Fcn44/1
  Sum11/1 -> Transfer Fcn21/1, Transfer Fcn20/1
  Transfer Fcn42/1 -> Sum20/1
  Sum1/1 -> Transfer Fcn2/1, Transfer Fcn1/1
  Sum15/1 -> Transfer Fcn36/1, Transfer Fcn35/1
  Transfer Fcn27/1 -> Sum22/2
  Transfer Fcn24/1 -> Sum16/2
  Transfer Fcn31/1 -> Sum14/1
  Transfer Fcn23/1 -> Sum16/1
  Sum14/1 -> Transfer Fcn33/1, Transfer Fcn32/1
  Sum23/1 -> Transfer Fcn27/1, Transfer Fcn31/1
  Transfer Fcn40/1 -> Sum19/1
  Sum16/1 -> Transfer Fcn38/1, Transfer Fcn37/1
  Transfer Fcn22/1 -> Sum13/1
  Transfer Fcn34/1 -> Sum12/2
  Transfer Fcn37/1 -> Sum17/1
  Transfer Fcn33/1 -> Sum23/2
  Transfer Fcn41/1 -> Sum17/2
  Sum4/1 -> Transfer Fcn7/1, Transfer Fcn6/1
  Transfer Fcn36/1 -> Sum14/2
  Sum10/1 -> Transfer Fcn19/1, Transfer Fcn18/1
  Sum22/1 -> Transfer Fcn30/1, Transfer Fcn29/1
  Transfer Fcn6/1 -> Sum5/1
  Transfer Fcn29/1 -> Sum23/1
  Transfer Fcn2/1 -> Sum/2
  Transfer Fcn28/1 -> Sum20/2
  Transfer Fcn17/1 -> Sum10/1
  Transfer Fcn30/1 -> Sum21/2
  Transfer Fcn43/1 -> Sum18/2
  Transfer Fcn5/1 -> Sum4/1
  Sum19/1 -> Transfer Fcn43/1, Transfer Fcn42/1
  Sum3/1 -> Transfer Fcn10/1, Transfer Fcn5/1
  Transfer Fcn32/1 -> Sum15/1
  Sum6/1 -> Sum5/2, Transfer Fcn11/1
  Transfer Fcn/1 -> Sum1/1
  Transfer Fcn21/1 -> Sum10/2
  Sum5/1 -> Transfer Fcn9/1, Transfer Fcn8/1
  Transfer Fcn7/1 -> Sum3/2
  Transfer Fcn4/1 -> Sum1/2
  Transfer Fcn11/1 -> Sum7/1
  Transfer Fcn10/1 -> Sum2/2
  Transfer Fcn3/1 -> Sum3/1
  Transfer Fcn8/1 -> Sum6/1
  Transfer Fcn19/1 -> Sum9/2
  Sum/1 -> Transfer Fcn/1
  Gain/1 -> Y/1
  U/1 -> Sum/1

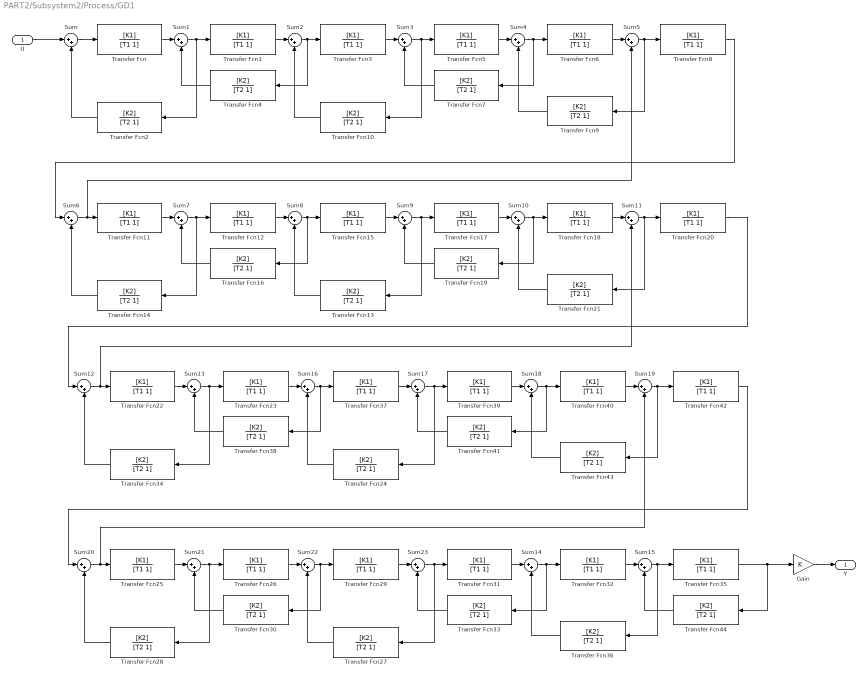
== system PART2/Subsystem2/Process/GD1 ==
  U : Inport
  Gain : Gain  Gain=K
  Sum{,1..23} (24 alike) : Sum  Inputs=|++
  Transfer Fcn{,1,3,5..6,8,11..12,15,17..18,20,22..23,25..26,29,31..32,35,37,39..40,42} (24 alike) : TransferFcn  Numerator=[K1]  Denominator=[T1 1]
  Transfer Fcn{2,4,7,9..10,13..14,16,19,21,24,27..28,30,33..34,36,38,41,43..44} (21 alike) : TransferFcn  Numerator=[K2]  Denominator=[T2 1]
  Y : Outport
  wires:
  Transfer Fcn14/1 -> Sum6/2
  Transfer Fcn13/1 -> Sum8/2
  Transfer Fcn18/1 -> Sum11/1
  Transfer Fcn1/1 -> Sum2/1
  Sum18/1 -> Transfer Fcn41/1, Transfer Fcn40/1
  Sum21/1 -> Transfer Fcn28/1, Transfer Fcn26/1
  Transfer Fcn26/1 -> Sum22/1
  Transfer Fcn15/1 -> Sum9/1
  Sum13/1 -> Transfer Fcn34/1, Transfer Fcn23/1
  Sum7/1 -> Transfer Fcn14/1, Transfer Fcn12/1
  Sum8/1 -> Transfer Fcn16/1, Transfer Fcn15/1
  Transfer Fcn20/1 -> Sum12/1
  Sum20/1 -> Sum19/2, Transfer Fcn25/1
  Transfer Fcn9/1 -> Sum4/2
  Transfer Fcn25/1 -> Sum21/1
  Sum12/1 -> Sum11/2, Transfer Fcn22/1
  Transfer Fcn12/1 -> Sum8/1
  Transfer Fcn16/1 -> Sum7/2
  Transfer Fcn44/1 -> Sum15/2
  Transfer Fcn39/1 -> Sum18/1
  Sum2/1 -> Transfer Fcn4/1, Transfer Fcn3/1
  Transfer Fcn38/1 -> Sum13/2
  Sum17/1 -> Transfer Fcn24/1, Transfer Fcn39/1
  Sum9/1 -> Transfer Fcn13/1, Transfer Fcn17/1
  Transfer Fcn35/1 -> Gain/1, Transfer Fcn44/1
  Sum11/1 -> Transfer Fcn21/1, Transfer Fcn20/1
  Transfer Fcn42/1 -> Sum20/1
  Sum1/1 -> Transfer Fcn2/1, Transfer Fcn1/1
  Sum15/1 -> Transfer Fcn36/1, Transfer Fcn35/1
  Transfer Fcn27/1 -> Sum22/2
  Transfer Fcn24/1 -> Sum16/2
  Transfer Fcn31/1 -> Sum14/1
  Transfer Fcn23/1 -> Sum16/1
  Sum14/1 -> Transfer Fcn33/1, Transfer Fcn32/1
  Sum23/1 -> Transfer Fcn27/1, Transfer Fcn31/1
  Transfer Fcn40/1 -> Sum19/1
  Sum16/1 -> Transfer Fcn38/1, Transfer Fcn37/1
  Transfer Fcn22/1 -> Sum13/1
  Transfer Fcn34/1 -> Sum12/2
  Transfer Fcn37/1 -> Sum17/1
  Transfer Fcn33/1 -> Sum23/2
  Transfer Fcn41/1 -> Sum17/2
  Sum4/1 -> Transfer Fcn7/1, Transfer Fcn6/1
  Transfer Fcn36/1 -> Sum14/2
  Sum10/1 -> Transfer Fcn19/1, Transfer Fcn18/1
  Sum22/1 -> Transfer Fcn30/1, Transfer Fcn29/1
  Transfer Fcn6/1 -> Sum5/1
  Transfer Fcn29/1 -> Sum23/1
  Transfer Fcn2/1 -> Sum/2
  Transfer Fcn28/1 -> Sum20/2
  Transfer Fcn17/1 -> Sum10/1
  Transfer Fcn30/1 -> Sum21/2
  Transfer Fcn43/1 -> Sum18/2
  Transfer Fcn5/1 -> Sum4/1
  Sum19/1 -> Transfer Fcn43/1, Transfer Fcn42/1
  Sum3/1 -> Transfer Fcn10/1, Transfer Fcn5/1
  Transfer Fcn32/1 -> Sum15/1
  Sum6/1 -> Sum5/2, Transfer Fcn11/1
  Transfer Fcn/1 -> Sum1/1
  Transfer Fcn21/1 -> Sum10/2
  Sum5/1 -> Transfer Fcn9/1, Transfer Fcn8/1
  Transfer Fcn7/1 -> Sum3/2
  Transfer Fcn4/1 -> Sum1/2
  Transfer Fcn11/1 -> Sum7/1
  Transfer Fcn10/1 -> Sum2/2
  Transfer Fcn3/1 -> Sum3/1
  Transfer Fcn8/1 -> Sum6/1
  Transfer Fcn19/1 -> Sum9/2
  Sum/1 -> Transfer Fcn/1
  Gain/1 -> Y/1
  U/1 -> Sum/1
